simulink model "propPDcontroller"  (R2021b)
settings: Solver=VariableStepAuto  StartTime=0.0  StopTime=200  RelTol=1e-3
settings Model: Creator=mluser  LastModifiedBy=mluser

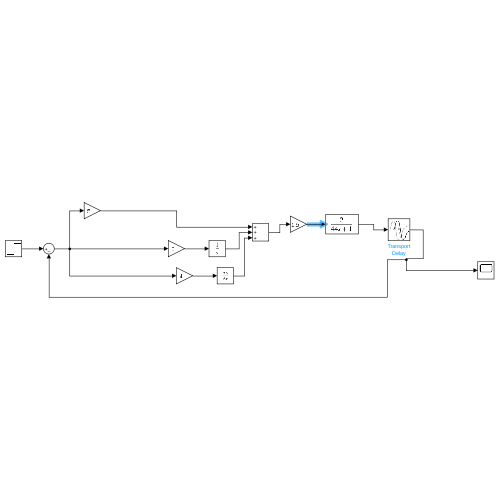
[thumbnail: Simulink's stored preview of the top-level diagram]
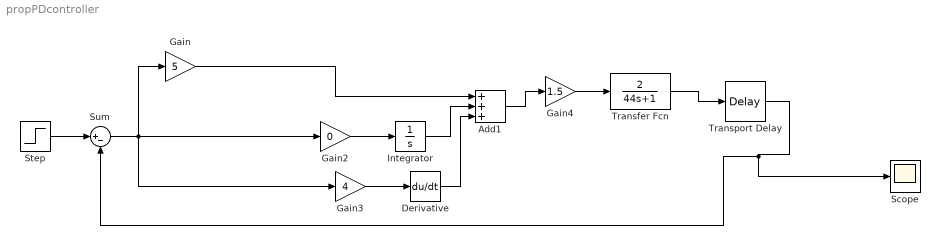
== system propPDcontroller ==
  Add1 : Sum  Inputs=+++
  Derivative : Derivative
  Gain : Gain  Gain=5
  Gain2 : Gain  Gain=0
  Gain3 : Gain  Gain=4
  Gain4 : Gain  Gain=1.5
  Integrator : Integrator
  Scope : Scope
  Step : Step  Before=1  SampleTime=0.0001
  Sum : Sum  Inputs=|+-
  Transfer Fcn : TransferFcn  Numerator=[2]  Denominator=[44 1]
  Transport Delay : TransportDelay
  wires:
  Step/1 -> Sum/1
  Sum/1 -> Gain3/1, Gain/1, Gain2/1
  Integrator/1 -> Add1/2
  Derivative/1 -> Add1/3
  Gain2/1 -> Integrator/1
  Gain3/1 -> Derivative/1
  Transfer Fcn/1 -> Transport Delay/1
  Transport Delay/1 -> Sum/2, Scope/1
  Gain/1 -> Add1/1
  Add1/1 -> Gain4/1
  Gain4/1 -> Transfer Fcn/1
